simulink library "motohawk_engine_lib"  (Simulink 6.3)
undefined symbols (not defined in the file or in its folder): cast_val, IndPowerMax, InjSequence, lookup_group, MAF_Sensor_p, motohawk_tex, motohawk_vardec_config_group, motohawk_vardec_path, SampleTime, SparkSequence, SteadyStateECT, txtTitle, WarmUpTimeConst
libraries: MotoHawk_lib x234, motohawk_annotations_lib x22, motohawk_control_primitives_lib x20, motohawk_engine_lib x8, motohawk_control_primitives_lib_new x3
(part 7 of 7)

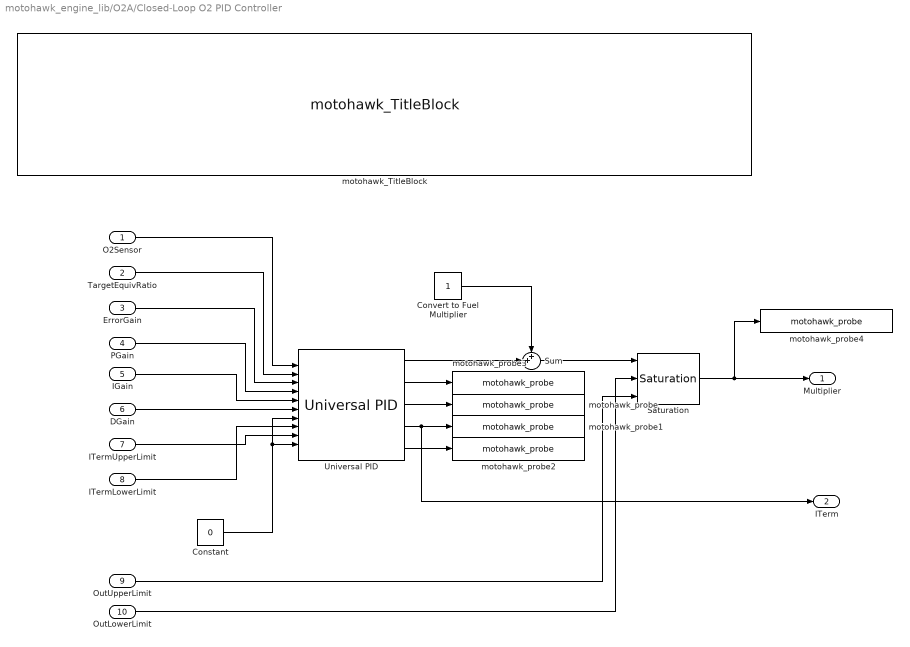
== system motohawk_engine_lib/O2A/Closed-Loop O2 PID Controller ==
  O2Sensor : Inport
  TargetEquivRatio : Inport  Port=2
  ErrorGain : Inport  Port=3
  PGain : Inport  Port=4
  IGain : Inport  Port=5
  DGain : Inport  Port=6
  ITermUpperLimit : Inport  Port=7
  ITermLowerLimit : Inport  Port=8
  OutUpperLimit : Inport  Port=9
  OutLowerLimit : Inport  Port=10
  Constant : Constant  Value=0
  Convert to Fuel Multiplier : Constant
  Saturation : motohawk_control_primitives_lib/Saturation
  Sum : Sum  Inputs=++|  SaturateOnIntegerOverflow=on  InputSameDT=on
  Universal PID : motohawk_control_primitives_lib/Universal PID  Description=|  samp_time=-1
      | /* Name: ErrorGain Unit:mult ClassID:VAR StorageID:FLASH Access:RW4+RW3+NA2+NA1 TypeID:UINT4                   
      |    Gain:0.000000001 Min:0.000000000 Max:4.000000000 Format:10.9 UpdateID:REMOTE Help:"This gain is applied to "
      |    "the error term before it is used to calculate the P, I and D terms." VardecSig:6C */                       
      |                                                                                                                
      | /* Name: ITermLowerLim Unit:0 ClassID:VAR StorageID:FLASH Access:RW4+RW3+NA2+NA1 TypeID:SINT2 Gain:0.1         
      |    Min:-3276.8 Max:3276.7 Format:5.1 UpdateID:REMOTE Help:"Lower limit on the I-term value." VardecSig:6C */   
      |                                                                                                                
      | /* Name: ITermUpperLim ClassID:VAR StorageID:FLASH Access:RW4+RW3+NA2+NA1 TypeID:SINT2 Gain:0.1 Min:-3276.8    
      |    Max:3276.7 Format:5.1 UpdateID:REMOTE Help:"Upper limit on I-term value." VardecSig:6C */                   
      |                                                                                                                
      | /* Name: PIDOutLowerLim ClassID:VAR StorageID:FLASH Access:RW4+RW3+NA2+NA1 TypeID:SINT2 Gain:0.1               
      |    Min:-3276.8 Max:3276.7 Format:5.1 UpdateID:REMOTE Help:"Lower limit on PID output." VardecSig:6C */         
      |                                                                                                                
      | /* Name: PIDOutUpperLim ClassID:VAR StorageID:FLASH Access:RW4+RW3+NA2+NA1 TypeID:SINT2 Gain:0.1               
      |    Min:-3276.8 Max:3276.7 Format:3.1 UpdateID:REMOTE Help:"Upper limit on PID output." VardecSig:6C */
  motohawk_TitleBlock : motohawk_annotations_lib/motohawk_TitleBlock  BlockType_='Mototron_Title_Block'  ttl=[txtTitle '\newline\rmClosed-loop O2 Control - PID for Bank A']  copyright="'THE INFORMATION CONTAINED IN THIS\\newlineDRAWING IS THE SOLE PROPERTY OF\\newlineMOTOTRON.  ANY REPRODUCTION IN\\newline PART OR AS A WHOLE WITHOUT THE\\newlineWRITTEN PERMISSION OF MOTOTRON\\newline IS PROHIBITED.\\fontsize{16}\\rm\\copyright\\rm\\fontsize{10} 2005'"  address='\fontsize{22}\it\fontname{Arial Black}MotoTron Corporation \fontname{Arial}\fontsize{10}\newline505 Marion Road, Oshkosh, WI, 54901\newlinewww.mototron.com (734) 822-7700'  image_file='mh.jpg'  pretty_print=on  edit_text=[motohawk_tex(get_param(bdroot, 'Description')) '\rm\newline' motohawk_tex(get_param(gcs, 'Name'))]  edit_as=6
  motohawk_probe : MotoHawk_lib/Calibration & Probing Blocks/motohawk_probe  nam=['O2Control_PTerm' bank]  show_more=on  name_source=Use Parameter  read_level=1  view_as=Number  enum_struct={'Disabled', 'Enabled'}  vector_style=Wide Row  use_help_units=on  help=['Closed-loop O2 control P-Term, for bank ' bank]  units='mult'  use_header_enum=off  row_header_enum={}  col_header_enum={}  use_precision=off  precision=''  gain=1  offset=0  exp=1  use_mototune_group=on  mototune_group=display_group
  motohawk_probe1 : MotoHawk_lib/Calibration & Probing Blocks/motohawk_probe  nam=['O2Control_ITerm' bank]  show_more=on  name_source=Use Parameter  read_level=1  view_as=Number  enum_struct={'Disabled', 'Enabled'}  vector_style=Wide Row  use_help_units=on  help=['Closed-loop O2 control I-Term, for bank ' bank]  units='mult'  use_header_enum=off  row_header_enum={}  col_header_enum={}  use_precision=off  precision=''  gain=1  offset=0  exp=1  use_mototune_group=on  mototune_group=display_group
  motohawk_probe2 : MotoHawk_lib/Calibration & Probing Blocks/motohawk_probe  nam=['O2Control_DTerm' bank]  show_more=on  name_source=Use Parameter  read_level=1  view_as=Number  enum_struct={'Disabled', 'Enabled'}  vector_style=Wide Row  use_help_units=on  help=['Closed-loop O2 control D-Term, for bank ' bank]  units='mult'  use_header_enum=off  row_header_enum={}  col_header_enum={}  use_precision=off  precision=''  gain=1  offset=0  exp=1  use_mototune_group=on  mototune_group=display_group
  motohawk_probe3 : MotoHawk_lib/Calibration & Probing Blocks/motohawk_probe  nam=['O2Control_ErrorTerm' bank]  show_more=on  name_source=Use Parameter  read_level=1  view_as=Number  enum_struct={'Disabled', 'Enabled'}  vector_style=Wide Row  use_help_units=on  help=['Closed-loop O2 control error-term, for bank ' bank]  units='mult'  use_header_enum=off  row_header_enum={}  col_header_enum={}  use_precision=off  precision=''  gain=1  offset=0  exp=1  use_mototune_group=on  mototune_group=display_group
  motohawk_probe4 : MotoHawk_lib/Calibration & Probing Blocks/motohawk_probe  nam=['O2FuelMult' bank]  show_more=on  name_source=Use Parameter  read_level=1  view_as=Number  enum_struct={'Disabled', 'Enabled'}  vector_style=Wide Row  use_help_units=on  help=['Closed-loop O2 control fuel multiplier, for bank ' bank]  units='mult'  use_header_enum=off  row_header_enum={}  col_header_enum={}  use_precision=off  precision=''  gain=1  offset=0  exp=1  use_mototune_group=on  mototune_group=display_group
  Multiplier : Outport
  ITerm : Outport  Port=2
  wires:
  Universal PID/2 -> motohawk_probe3/1
  OutLowerLimit/1 -> Saturation/2
  ITermLowerLimit/1 -> Universal PID/8
  ITermUpperLimit/1 -> Universal PID/9
  Sum/1 -> Saturation/1
  Universal PID/1 -> Sum/2
  Convert to Fuel Multiplier/1 -> Sum/1
  OutUpperLimit/1 -> Saturation/3
  DGain/1 -> Universal PID/6
  IGain/1 -> Universal PID/5
  PGain/1 -> Universal PID/4
  ErrorGain/1 -> Universal PID/3
  TargetEquivRatio/1 -> Universal PID/2
  O2Sensor/1 -> Universal PID/1
  Saturation/1 -> motohawk_probe4/1, Multiplier/1
  Universal PID/5 -> motohawk_probe2/1
  Constant/1 -> Universal PID/7, Universal PID/10
  Universal PID/4 -> ITerm/1, motohawk_probe1/1
  Universal PID/3 -> motohawk_probe/1

== system motohawk_engine_lib/O2A/Equivalence Ratio Perturbation ==
  note: When low, switch to rich.
      | When high, switch to lean.
  O2Sensor : Inport
  DesEquivRatio : Inport  Port=2
  RichEquivRatioTargetDelta : Inport  Port=3
  LeanEquivRatioTargetDelta : Inport  Port=4
  RichEquivRatioSwPtDelta : Inport  Port=5
  LeanEquivRatioSwPtDelta : Inport  Port=6
  Hysteresis : Subsystem
  LT : RelationalOperator  ZeroCross=off  InputSameDT=on
  LT1 : RelationalOperator  Operator=<=  ZeroCross=off  InputSameDT=on
  Logical Operator : Logic  Operator=NOT
  Sum1 : Sum  SaturateOnIntegerOverflow=on
  Sum2 : Sum  Inputs=-+  SaturateOnIntegerOverflow=on
  Sum3 : Sum  SaturateOnIntegerOverflow=on
  Sum4 : Sum  Inputs=+-  SaturateOnIntegerOverflow=on
  Switch2 : Switch  Threshold=1  ZeroCross=off  InputSameDT=on
  motohawk_TitleBlock : motohawk_annotations_lib/motohawk_TitleBlock  BlockType_='Mototron_Title_Block'  ttl=[txtTitle '\newline\rmO2 Control Target Equivalence Ratio Perturbation around Stoichiometric']  copyright="'THE INFORMATION CONTAINED IN THIS\\newlineDRAWING IS THE SOLE PROPERTY OF\\newlineMOTOTRON.  ANY REPRODUCTION IN\\newline PART OR AS A WHOLE WITHOUT THE\\newlineWRITTEN PERMISSION OF MOTOTRON\\newline IS PROHIBITED.\\fontsize{16}\\rm\\copyright\\rm\\fontsize{10} 2005'"  address='\fontsize{22}\it\fontname{Arial Black}MotoTron Corporation \fontname{Arial}\fontsize{10}\newline505 Marion Road, Oshkosh, WI, 54901\newlinewww.mototron.com (734) 822-7700'  image_file='mh.jpg'  pretty_print=on  edit_text=[motohawk_tex(get_param(bdroot, 'Description')) '\rm\newline' motohawk_tex(get_param(gcs, 'Name'))]  edit_as=6
  motohawk_fault_def : MotoHawk_lib/Fault Management Blocks/motohawk_fault_def  nam=['O2FailedLean',bank]  mode=Enabled  id=[]  x=25  y=50  input_suspected=on  indeterminate=off  increment_xy=on  downsample_count=1  ovr_cals=on  ovr_actions=on  show_actions=off  action1_name=''  action1_cond=(None)  action2_name=''  action2_cond=(None)  action3_name=''  action3_cond=(None)  action4_name=''  action4_cond=(None)
  motohawk_fault_def1 : MotoHawk_lib/Fault Management Blocks/motohawk_fault_def  nam=['O2FailedRich',bank]  mode=Enabled  id=[]  x=25  y=50  input_suspected=on  indeterminate=off  increment_xy=on  downsample_count=1  ovr_cals=on  ovr_actions=on  show_actions=off  action1_name=''  action1_cond=(None)  action2_name=''  action2_cond=(None)  action3_name=''  action3_cond=(None)  action4_name=''  action4_cond=(None)
  Target Phi : Outport
  wires:
  Logical Operator/1 -> Switch2/2
  O2Sensor/1 -> LT/1, LT1/1
  Hysteresis/1("Out (Lo=0, Hi=1)") -> Logical Operator/1
  LT1/1 -> motohawk_fault_def/1, Hysteresis/2(Lo)  "BelowLean"
  LT/1 -> motohawk_fault_def1/1, Hysteresis/1(Hi)  "AboveRich"
  RichEquivRatioTargetDelta/1 -> Sum1/1
  LeanEquivRatioTargetDelta/1 -> Sum2/1
  Sum1/1 -> Switch2/1
  Sum2/1 -> Switch2/3
  LeanEquivRatioSwPtDelta/1 -> Sum4/2
  RichEquivRatioSwPtDelta/1 -> Sum3/2
  DesEquivRatio/1 -> Sum3/1, Sum4/1, Sum2/2, Sum1/2
  Switch2/1 -> Target Phi/1
  Sum4/1 -> LT1/2
  Sum3/1 -> LT/2

== system motohawk_engine_lib/O2A/O2 Calibrations ==
  Bus Creator : BusCreator  Inputs=12
  motohawk_TitleBlock : motohawk_annotations_lib/motohawk_TitleBlock  BlockType_='Mototron_Title_Block'  ttl=[txtTitle '\newline\rmClosed-Loop O2 Control Calibrations']  copyright="'THE INFORMATION CONTAINED IN THIS\\newlineDRAWING IS THE SOLE PROPERTY OF\\newlineMOTOTRON.  ANY REPRODUCTION IN\\newline PART OR AS A WHOLE WITHOUT THE\\newlineWRITTEN PERMISSION OF MOTOTRON\\newline IS PROHIBITED.\\fontsize{16}\\rm\\copyright\\rm\\fontsize{10} 2005'"  address='\fontsize{22}\it\fontname{Arial Black}MotoTron Corporation \fontname{Arial}\fontsize{10}\newline505 Marion Road, Oshkosh, WI, 54901\newlinewww.mototron.com (734) 822-7700'  image_file='mh.jpg'  pretty_print=on  edit_text=[motohawk_tex(get_param(bdroot, 'Description')) '\rm\newline' motohawk_tex(get_param(gcs, 'Name'))]  edit_as=6
  motohawk_calibration1 : MotoHawk_lib/Calibration & Probing Blocks/motohawk_calibration  nam=['LeanEquivRatioTargetDelta' bank]  val=.05  storage=Calibration  show_more=on  name_source=Use Parameter  data_type=Inherit from 'Default Value'  read_level=1  write_level=1  ovr_cals=on  view_as=Number  enum_struct={'Disabled', 'Enabled'}  vector_style=Wide Row  use_help_units=on  help='Target equivalence ratio below desired, when driving lean'  units='ratio'  use_header_enum=off  row_header_enum={}  col_header_enum={}  use_min_max=on  min_val=0  max_val=1.0  use_precision=off  precision=''  gain=1  offset=0  exp=1  use_mototune_group=on  mototune_group=cal_group
  motohawk_calibration10 : MotoHawk_lib/Calibration & Probing Blocks/motohawk_calibration  nam=['O2ControlOutUpperLimit',bank]  val=1.4  storage=Calibration  show_more=on  name_source=Use Parameter  data_type=Inherit from 'Default Value'  read_level=1  write_level=1  ovr_cals=on  view_as=Number  enum_struct={'Disabled', 'Enabled'}  vector_style=Wide Row  use_help_units=on  help='PID fuel multiplier output upper limit for closed-loop O2 control'  units='mult'  use_header_enum=off  row_header_enum={}  col_header_enum={}  use_min_max=on  min_val=-inf  max_val=inf  use_precision=off  precision=''  gain=1  offset=0  exp=1  use_mototune_group=on  mototune_group=cal_group
  motohawk_calibration11 : MotoHawk_lib/Calibration & Probing Blocks/motohawk_calibration  nam=['O2ControlOutLowerLimit',bank]  val=.6  storage=Calibration  show_more=on  name_source=Use Parameter  data_type=Inherit from 'Default Value'  read_level=1  write_level=1  ovr_cals=on  view_as=Number  enum_struct={'Disabled', 'Enabled'}  vector_style=Wide Row  use_help_units=on  help='PID fuel multiplier output lower limit for closed-loop O2 control'  units='mult'  use_header_enum=off  row_header_enum={}  col_header_enum={}  use_min_max=on  min_val=-inf  max_val=inf  use_precision=off  precision=''  gain=1  offset=0  exp=1  use_mototune_group=on  mototune_group=cal_group
  motohawk_calibration12 : MotoHawk_lib/Calibration & Probing Blocks/motohawk_calibration  nam=['RichEquivRatioTargetDelta' bank]  val=.05  storage=Calibration  show_more=on  name_source=Use Parameter  data_type=Inherit from 'Default Value'  read_level=1  write_level=1  ovr_cals=on  view_as=Number  enum_struct={'Disabled', 'Enabled'}  vector_style=Wide Row  use_help_units=on  help='Target equivalence ratio below desired, when driving lean'  units='ratio'  use_header_enum=off  row_header_enum={}  col_header_enum={}  use_min_max=on  min_val=0  max_val=1.0  use_precision=off  precision=''  gain=1  offset=0  exp=1  use_mototune_group=on  mototune_group=cal_group
  motohawk_calibration2 : MotoHawk_lib/Calibration & Probing Blocks/motohawk_calibration  nam=['RichEquivRatioSwPtDelta',bank]  val=.01  storage=Calibration  show_more=on  name_source=Use Parameter  data_type=Inherit from 'Default Value'  read_level=1  write_level=1  ovr_cals=on  view_as=Number  enum_struct={'Disabled', 'Enabled'}  vector_style=Wide Row  use_help_units=on  help='Switch point equivalence ratio above desired, when driving rich, and changing to lean'  units='ratio'  use_header_enum=off  row_header_enum={}  col_header_enum={}  use_min_max=on  min_val=0  max_val=1.0  use_precision=off  precision=''  gain=1  offset=0  exp=1  use_mototune_group=on  mototune_group=cal_group
  motohawk_calibration3 : MotoHawk_lib/Calibration & Probing Blocks/motohawk_calibration  nam=['LeanEquivRatioSwPtDelta',bank]  val=.01  storage=Calibration  show_more=on  name_source=Use Parameter  data_type=Inherit from 'Default Value'  read_level=1  write_level=1  ovr_cals=on  view_as=Number  enum_struct={'Disabled', 'Enabled'}  vector_style=Wide Row  use_help_units=on  help='Switch point equivalence ratio below desired, when driving lean, and changing to rich'  units='ratio'  use_header_enum=off  row_header_enum={}  col_header_enum={}  use_min_max=on  min_val=0  max_val=1.0  use_precision=off  precision=''  gain=1  offset=0  exp=1  use_mototune_group=on  mototune_group=cal_group
  motohawk_calibration4 : MotoHawk_lib/Calibration & Probing Blocks/motohawk_calibration  nam=['O2ControlErrorGain',bank]  val=.2  storage=Calibration  show_more=on  name_source=Use Parameter  data_type=Inherit from 'Default Value'  read_level=1  write_level=1  ovr_cals=on  view_as=Number  enum_struct={'Disabled', 'Enabled'}  vector_style=Wide Row  use_help_units=on  help='PID error gain for closed-loop O2 control'  units='mult'  use_header_enum=off  row_header_enum={}  col_header_enum={}  use_min_max=on  min_val=-inf  max_val=inf  use_precision=off  precision=''  gain=1  offset=0  exp=1  use_mototune_group=on  mototune_group=cal_group
  motohawk_calibration5 : MotoHawk_lib/Calibration & Probing Blocks/motohawk_calibration  nam=['O2ControlPGain',bank]  val=1  storage=Calibration  show_more=on  name_source=Use Parameter  data_type=Inherit from 'Default Value'  read_level=1  write_level=1  ovr_cals=on  view_as=Number  enum_struct={'Disabled', 'Enabled'}  vector_style=Wide Row  use_help_units=on  help='PID P-Term gain for closed-loop O2 control'  units='mult'  use_header_enum=off  row_header_enum={}  col_header_enum={}  use_min_max=on  min_val=-inf  max_val=inf  use_precision=off  precision=''  gain=1  offset=0  exp=1  use_mototune_group=on  mototune_group=cal_group
  motohawk_calibration6 : MotoHawk_lib/Calibration & Probing Blocks/motohawk_calibration  nam=['O2ControlIGain',bank]  val=2  storage=Calibration  show_more=on  name_source=Use Parameter  data_type=Inherit from 'Default Value'  read_level=1  write_level=1  ovr_cals=on  view_as=Number  enum_struct={'Disabled', 'Enabled'}  vector_style=Wide Row  use_help_units=on  help='PID I-Term gain for closed-loop O2 control'  units='mult'  use_header_enum=off  row_header_enum={}  col_header_enum={}  use_min_max=on  min_val=-inf  max_val=inf  use_precision=off  precision=''  gain=1  offset=0  exp=1  use_mototune_group=on  mototune_group=cal_group
  motohawk_calibration7 : MotoHawk_lib/Calibration & Probing Blocks/motohawk_calibration  nam=['O2ControlDGain',bank]  val=0  storage=Calibration  show_more=on  name_source=Use Parameter  data_type=Inherit from 'Default Value'  read_level=1  write_level=1  ovr_cals=on  view_as=Number  enum_struct={'Disabled', 'Enabled'}  vector_style=Wide Row  use_help_units=on  help='PID D-Term gain for closed-loop O2 control'  units='mult'  use_header_enum=off  row_header_enum={}  col_header_enum={}  use_min_max=on  min_val=-inf  max_val=inf  use_precision=off  precision=''  gain=1  offset=0  exp=1  use_mototune_group=on  mototune_group=cal_group
  motohawk_calibration8 : MotoHawk_lib/Calibration & Probing Blocks/motohawk_calibration  nam=['O2ControlITermLowerLimit',bank]  val=-.4  storage=Calibration  show_more=on  name_source=Use Parameter  data_type=Inherit from 'Default Value'  read_level=1  write_level=1  ovr_cals=on  view_as=Number  enum_struct={'Disabled', 'Enabled'}  vector_style=Wide Row  use_help_units=on  help='PID I-Term lower limit for closed-loop O2 control'  units='mult'  use_header_enum=off  row_header_enum={}  col_header_enum={}  use_min_max=on  min_val=-inf  max_val=inf  use_precision=off  precision=''  gain=1  offset=0  exp=1  use_mototune_group=on  mototune_group=cal_group
  motohawk_calibration9 : MotoHawk_lib/Calibration & Probing Blocks/motohawk_calibration  nam=['O2ControlITermUpperLimit',bank]  val=.3  storage=Calibration  show_more=on  name_source=Use Parameter  data_type=Inherit from 'Default Value'  read_level=1  write_level=1  ovr_cals=on  view_as=Number  enum_struct={'Disabled', 'Enabled'}  vector_style=Wide Row  use_help_units=on  help='PID I-Term upper limit for closed-loop O2 control'  units='mult'  use_header_enum=off  row_header_enum={}  col_header_enum={}  use_min_max=on  min_val=-inf  max_val=inf  use_precision=off  precision=''  gain=1  offset=0  exp=1  use_mototune_group=on  mototune_group=cal_group
  Calibrations : Outport
  wires:
  motohawk_calibration12/1 -> Bus Creator/1  "RichEquivRatioTargetDelta"
  Bus Creator/1 -> Calibrations/1
  motohawk_calibration11/1 -> Bus Creator/12  "O2ControlOutLowerLimit"
  motohawk_calibration10/1 -> Bus Creator/11  "O2ControlOutUpperLimit"
  motohawk_calibration8/1 -> Bus Creator/10  "O2ControlItermLowerLimit"
  motohawk_calibration9/1 -> Bus Creator/9  "O2ControlITermUpperLimit"
  motohawk_calibration7/1 -> Bus Creator/8  "O2ControlDGain"
  motohawk_calibration6/1 -> Bus Creator/7  "O2ControlIGain"
  motohawk_calibration5/1 -> Bus Creator/6  "O2ControlPGain"
  motohawk_calibration4/1 -> Bus Creator/5  "O2ControlErrorGain"
  motohawk_calibration3/1 -> Bus Creator/4  "LeanEquivRatioSwPtDelta"
  motohawk_calibration2/1 -> Bus Creator/3  "RichEquivRatioSwPtDelta"
  motohawk_calibration1/1 -> Bus Creator/2  "LeanEquivRatioTargetDelta"

== system motohawk_engine_lib/Speed Density - MAP Referenced/C to K1 ==
  C : Inport
  C to K : Fcn  Expr=u(1) + 273.2
  K : Outport
  wires:
  C/1 -> C to K/1
  C to K/1 -> K/1

== system motohawk_engine_lib/Speed Density - MAP Referenced - Adaptive/Adapt Volumetric Efficiency ==
  SSEngOpr [bool] : Inport
  MAF_Sensor [g/s] : Inport  Port=2
  MAF_Model [g/s] : Inport  Port=3
  Abs : Abs  SaturateOnIntegerOverflow=on
  Adapt VolEff Map : Subsystem
  Logical Operator : Logic  Inputs=3
  Product0 : Product  SaturateOnIntegerOverflow=on  InputSameDT=on
  Relational Operator : RelationalOperator  Operator=<=  InputSameDT=on
  Safe Divide : Subsystem
  Sum1 : Sum  Inputs=+-  SaturateOnIntegerOverflow=on  InputSameDT=on
  motohawk_TitleBlock : motohawk_annotations_lib/motohawk_TitleBlock  BlockType_='Mototron_Title_Block'  ttl=[txtTitle '\newline\rmDetermine whether to adapt the volumetric efficiency map\newlineand compute the error for modifying the map']  copyright="'THE INFORMATION CONTAINED IN THIS\\newlineDRAWING IS THE SOLE PROPERTY OF\\newlineMOTOTRON.  ANY REPRODUCTION IN\\newline PART OR AS A WHOLE WITHOUT THE\\newlineWRITTEN PERMISSION OF MOTOTRON\\newline IS PROHIBITED.\\fontsize{16}\\rm\\copyright\\rm\\fontsize{10} 2005'"  address='\fontsize{22}\it\fontname{Arial Black}MotoTron Corporation \fontname{Arial}\fontsize{10}\newline505 Marion Road, Oshkosh, WI, 54901\newlinewww.mototron.com (734) 822-7700'  image_file='mh.jpg'  pretty_print=on  edit_text=[motohawk_tex(get_param(bdroot, 'Description')) '\rm\newline' motohawk_tex(get_param(gcs, 'Name'))]  edit_as=6
  motohawk_calibration : MotoHawk_lib/Calibration & Probing Blocks/motohawk_calibration  nam='VEAdaptEnable'  val=false  storage=Display  show_more=on  name_source=Use Parameter  data_type=Inherit from 'Default Value'  read_level=1  write_level=1  ovr_cals=on  view_as=Enumeration  enum_struct={'Disabled', 'Enabled'}  vector_style=Wide Row  use_help_units=on  help='Determines whether the Volumetric Efficiency map will be adapted using the MAF sensor'  units='bool'  use_header_enum=off  row_header_enum={}  col_header_enum={}  use_min_max=off  min_val=-inf  max_val=inf  use_precision=off  precision=''  gain=1  offset=0  exp=1  use_mototune_group=on  mototune_group=lookup_group(gcb)
  motohawk_calibration1 : MotoHawk_lib/Calibration & Probing Blocks/motohawk_calibration  nam='VEAdaptDelta'  val=VEAdaptDelta  storage=Calibration  show_more=on  name_source=Use Parameter  data_type=Inherit from 'Default Value'  read_level=1  write_level=1  ovr_cals=on  view_as=Number  enum_struct={'Disabled', 'Enabled'}  vector_style=Wide Row  use_help_units=on  help='VolEff_Error must be less than this delta to adapt the VolEff map'  units='mult'  use_header_enum=off  row_header_enum={}  col_header_enum={}  use_min_max=on  min_val=0  max_val=2  use_precision=off  precision=''  gain=1  offset=0  exp=1  use_mototune_group=on  mototune_group=lookup_group(gcb)
  motohawk_calibration2 : MotoHawk_lib/Calibration & Probing Blocks/motohawk_calibration  nam='VEAdaptGain'  val=VEAdaptGain  storage=Calibration  show_more=on  name_source=Use Parameter  data_type=Inherit from 'Default Value'  read_level=1  write_level=1  ovr_cals=on  view_as=Number  enum_struct={'Disabled', 'Enabled'}  vector_style=Wide Row  use_help_units=on  help="'Gain for updating VE table.  This fraction of the error is added to the map every 5ms.'"  units=''  use_header_enum=off  row_header_enum={}  col_header_enum={}  use_min_max=on  min_val=0  max_val=1  use_precision=off  precision='8.6'  gain=1  offset=0  exp=1  use_mototune_group=on  mototune_group=lookup_group(gcb)
  motohawk_probe1 : MotoHawk_lib/Calibration & Probing Blocks/motohawk_probe  nam='VolEff_Error'  show_more=on  name_source=Use Parameter  read_level=1  view_as=Number  enum_struct={'Disabled', 'Enabled'}  vector_style=Wide Row  use_help_units=on  help='Error in Volumetric Efficiency at the current operating point, as compared to MAF sensor'  units=''  use_header_enum=off  row_header_enum={}  col_header_enum={}  use_precision=off  precision=''  gain=1  offset=0  exp=1  use_mototune_group=on  mototune_group=lookup_group(gcb)
  motohawk_probe2 : MotoHawk_lib/Calibration & Probing Blocks/motohawk_probe  nam='MAF_ModelError'  show_more=on  name_source=Use Parameter  read_level=1  view_as=Number  enum_struct={'Disabled', 'Enabled'}  vector_style=Wide Row  use_help_units=on  help='Air Mass Flow Rate error, as compared to MAF sensor'  units='g/s'  use_header_enum=off  row_header_enum={}  col_header_enum={}  use_precision=off  precision=''  gain=1  offset=0  exp=1  use_mototune_group=on  mototune_group=lookup_group(gcb)
  motohawk_probe3 : MotoHawk_lib/Calibration & Probing Blocks/motohawk_probe  nam='VEAdapting'  show_more=on  name_source=Use Parameter  read_level=1  view_as=Enumeration  enum_struct={'Not adapting', 'Adapting'}  vector_style=Wide Row  use_help_units=on  help='Indicates whether the volumetric efficiency map is currently being adjusted'  units=''  use_header_enum=off  row_header_enum={}  col_header_enum={}  use_precision=off  precision=''  gain=1  offset=0  exp=1  use_mototune_group=on  mototune_group=lookup_group(gcb)
  wires:
  Product0/1 -> Adapt VolEff Map/1(error)
  motohawk_calibration2/1 -> Product0/2
  MAF_Model [g/s]/1 -> Safe Divide/2(Inport), Sum1/2
  MAF_Sensor [g/s]/1 -> Sum1/1
  Sum1/1 -> Safe Divide/1(X), motohawk_probe2/1
  Safe Divide/1(" ") -> Abs/1, motohawk_probe1/1, Product0/1
  motohawk_calibration1/1 -> Relational Operator/2
  Relational Operator/1 -> Logical Operator/3
  Abs/1 -> Relational Operator/1
  SSEngOpr [bool]/1 -> Logical Operator/2
  Logical Operator/1 -> motohawk_probe3/1, Adapt VolEff Map/Enable
  motohawk_calibration/1 -> Logical Operator/1

== system motohawk_engine_lib/Speed Density - MAP Referenced - Adaptive/C to K1 ==
  C : Inport
  C to K : Fcn  Expr=u(1) + 273.2
  K : Outport
  wires:
  C to K/1 -> K/1
  C/1 -> C to K/1

== system motohawk_engine_lib/Subsystem/Enabled Subsystem ==
  In1 : Inport
  Enable : EnablePort  StatesWhenEnabling=reset
  Out1 : Outport  OutputWhenDisabled=reset  InitialOutput=0
  wires:
  In1/1 -> Out1/1

== system motohawk_engine_lib/Idle Governor/Idle State Determination/Determine if RPM is Falling ==
  note: Determine whether RPM is falling
  RPM : Inport
  Derivitive : motohawk_control_primitives_lib/Derivitive  samp_time=-1
  Falling RPM is Negative Derivative : Gain  Gain=-1
  Median Filter : motohawk_control_primitives_lib/Median Filter  buffer_size=17
  Relational Operator : RelationalOperator  Operator=<
  motohawk_calibration : MotoHawk_lib/Calibration & Probing Blocks/motohawk_calibration  nam='RPMFallingRate'  val=4  storage=Calibration  show_more=on  name_source=Use Parameter  data_type=Inherit from 'Default Value'  read_level=1  write_level=1  ovr_cals=on  view_as=Number  enum_struct={'Disabled', 'Enabled'}  vector_style=Wide Row  use_help_units=on  help='The minimum rate of change in RPM that triggers RPMFalling - This should be a positive value'  units='RPM/sec'  use_header_enum=off  row_header_enum={}  col_header_enum={}  use_min_max=on  min_val=0  max_val=1000  use_precision=off  precision=''  gain=1  offset=0  exp=1  use_mototune_group=off  mototune_group=motohawk_vardec_path(gcb)
  motohawk_probe : MotoHawk_lib/Calibration & Probing Blocks/motohawk_probe  nam='RPMFalling'  show_more=off  name_source=Use Parameter  read_level=1  view_as=Number  enum_struct={'Disabled', 'Enabled'}  vector_style=Wide Row  use_help_units=off  help=''  units=''  use_header_enum=off  row_header_enum={}  col_header_enum={}  use_precision=off  precision=''  gain=1  offset=0  exp=1  use_mototune_group=off  mototune_group=motohawk_vardec_path(gcb)
  RPM Falling : Outport
  wires:
  Falling RPM is Negative Derivative/1 -> Relational Operator/2
  RPM/1 -> Derivitive/1
  Relational Operator/1 -> RPM Falling/1, motohawk_probe/1
  motohawk_calibration/1 -> Falling RPM is Negative Derivative/1
  Median Filter/1 -> Relational Operator/1
  Derivitive/1 -> Median Filter/1

== system motohawk_engine_lib/Linear Sensor Characterization w Adapt/ADAPT SCALING/ADAPT HI ==
  ADAPT_REQUEST : Inport
  ADAPT_ENABLE : Inport  Port=2
  CUR_ADAPT_PT : Inport  Port=3
  ADAPT_RANGE_MAX : Inport  Port=4
  ADAPT_RANGE_MIN : Inport  Port=5
  ADAPT_MIN_DELTA : Inport  Port=6
  MAX_LAST5 : Inport  Port=7
  Abs : Abs  SaturateOnIntegerOverflow=on
  Data Type Conversion : DataTypeConversion  OutDataTypeMode=double  SaturateOnIntegerOverflow=on  RndMeth=Zero
  Logical Operator1 : Logic  Inputs=5  AllPortsSameDT=off
  Logical Operator2 : Logic  Operator=OR  AllPortsSameDT=off
  Logical Operator4 : Logic  Inputs=4  AllPortsSameDT=off
  Relational Operator3 : RelationalOperator  Operator=>  LogicOutDataTypeMode=Boolean
  Relational Operator5 : RelationalOperator  Operator=<=  LogicOutDataTypeMode=Boolean
  Relational Operator6 : RelationalOperator  LogicOutDataTypeMode=Boolean
  Relational Operator9 : RelationalOperator  Operator=>  LogicOutDataTypeMode=Boolean
  Store Current Position : Subsystem  TreatAsAtomicUnit=on
  Sum2 : Sum  Inputs=|+-  SaturateOnIntegerOverflow=on
  ADAPTED_ENDPT : Outport
  wires:
  ADAPT_REQUEST/1 -> Logical Operator4/4
  Logical Operator4/1 -> Logical Operator2/2
  MAX_LAST5/1 -> Relational Operator6/1, Relational Operator5/1, Relational Operator9/1, Store Current Position/1(IN_FILT), Sum2/1
  ADAPT_ENABLE/1 -> Logical Operator4/3, Logical Operator1/4
  Data Type Conversion/1 -> Sum2/2, Relational Operator9/2, ADAPTED_ENDPT/1
  ADAPT_MIN_DELTA/1 -> Relational Operator3/2
  Abs/1 -> Relational Operator3/1
  Relational Operator3/1 -> Logical Operator1/5
  Sum2/1 -> Abs/1
  CUR_ADAPT_PT/1 -> Data Type Conversion/1
  Relational Operator9/1 -> Logical Operator1/1
  Relational Operator5/1 -> Logical Operator4/1, Logical Operator1/2
  Relational Operator6/1 -> Logical Operator4/2, Logical Operator1/3
  ADAPT_RANGE_MAX/1 -> Relational Operator5/2
  ADAPT_RANGE_MIN/1 -> Relational Operator6/2
  Logical Operator1/1 -> Logical Operator2/1
  Logical Operator2/1 -> Store Current Position/Enable

== system motohawk_engine_lib/Linear Sensor Characterization w Adapt/ADAPT SCALING/ADAPT LO ==
  ADAPT_REQUEST : Inport
  ADAPT_ENABLE : Inport  Port=2
  CUR_ADAPT_PT : Inport  Port=3
  ADAPT_RANGE_MAX : Inport  Port=4
  ADAPT_RANGE_MIN : Inport  Port=5
  ADAPT_MIN_DELTA : Inport  Port=6
  MAX_LAST5 : Inport  Port=7
  Abs : Abs  SaturateOnIntegerOverflow=on
  Data Type Conversion : DataTypeConversion  OutDataTypeMode=double  SaturateOnIntegerOverflow=on  RndMeth=Zero
  Logical Operator1 : Logic  Inputs=5  AllPortsSameDT=off
  Logical Operator2 : Logic  Operator=OR  AllPortsSameDT=off
  Logical Operator4 : Logic  Inputs=4  AllPortsSameDT=off
  Relational Operator3 : RelationalOperator  Operator=>  LogicOutDataTypeMode=Boolean
  Relational Operator5 : RelationalOperator  Operator=<=  LogicOutDataTypeMode=Boolean
  Relational Operator6 : RelationalOperator  LogicOutDataTypeMode=Boolean
  Relational Operator9 : RelationalOperator  Operator=<  LogicOutDataTypeMode=Boolean
  Store Current Position : Subsystem  TreatAsAtomicUnit=on
  Sum2 : Sum  Inputs=|+-  SaturateOnIntegerOverflow=on
  ADAPTED_ENDPT : Outport
  wires:
  Logical Operator4/1 -> Logical Operator2/2
  ADAPT_REQUEST/1 -> Logical Operator4/4
  Logical Operator2/1 -> Store Current Position/Enable
  Logical Operator1/1 -> Logical Operator2/1
  ADAPT_RANGE_MIN/1 -> Relational Operator6/2
  ADAPT_RANGE_MAX/1 -> Relational Operator5/2
  Relational Operator6/1 -> Logical Operator4/2, Logical Operator1/3
  Relational Operator5/1 -> Logical Operator4/1, Logical Operator1/2
  Relational Operator9/1 -> Logical Operator1/1
  CUR_ADAPT_PT/1 -> Data Type Conversion/1
  Sum2/1 -> Abs/1
  Relational Operator3/1 -> Logical Operator1/5
  Abs/1 -> Relational Operator3/1
  ADAPT_MIN_DELTA/1 -> Relational Operator3/2
  Data Type Conversion/1 -> ADAPTED_ENDPT/1, Relational Operator9/2, Sum2/2
  ADAPT_ENABLE/1 -> Logical Operator4/3, Logical Operator1/4
  MAX_LAST5/1 -> Sum2/1, Store Current Position/1(IN_FILT), Relational Operator9/1, Relational Operator5/1, Relational Operator6/1

== system motohawk_engine_lib/Linear Sensor Characterization w Adapt/ADAPT SCALING/MinMaxFilter ==
  Input : Inport
  Bus Creator : BusCreator  Inputs=2
  MinMax : MinMax  Function=max  Inputs=5  SaturateOnIntegerOverflow=on  InputSameDT=on
  MinMax1 : MinMax  Inputs=5  SaturateOnIntegerOverflow=on  InputSameDT=on
  Unit Delay{,1,3..4} (4 alike) : UnitDelay  SampleTime=-1
  Min_Max : Outport
  wires:
  Input/1 -> Unit Delay4/1, MinMax/1, MinMax1/5
  MinMax1/1 -> Bus Creator/2  "min_last5"
  MinMax/1 -> Bus Creator/1  "max_last5"
  Unit Delay1/1 -> MinMax1/1, MinMax/5
  Unit Delay/1 -> MinMax1/2, Unit Delay1/1, MinMax/4
  Unit Delay3/1 -> Unit Delay/1, MinMax1/3, MinMax/3
  Unit Delay4/1 -> Unit Delay3/1, MinMax1/4, MinMax/2
  Bus Creator/1 -> Min_Max/1

== system motohawk_engine_lib/Model Fuel Puddle Mass/Enabled Tau-X Algorithm/Tau-X Fuel Model ==
  note: Tau - Puddle evaporation time constant
      | X - Fraction of fuel injected that adds to the puddle
  note: Puddle mass is modeled by integrating
      | the difference between the desired fuel rate
      | and the actual fuel rate
  Fdes [g/s] : Inport
  X [frac] : Inport  Port=2
  Tau [1/s] : Inport  Port=3
  MaxPuddle [mg] : Inport  Port=4
  InitPuddle [mg] : Inport  Port=5
  Can't Have Negative Puddle Mass1 : Constant  Value=0
  Can't have negative puddle mass : Constant  Value=0
  Can't inject negative fuel : MinMax  Function=max  Inputs=2  SaturateOnIntegerOverflow=on  InputSameDT=on
  Compute using grams : Gain  Orientation=left  Gain=1/1000  SaturateOnIntegerOverflow=on
  Initialize puddle mass on first sample : motohawk_control_primitives_lib/First Time
  Integrator : motohawk_control_primitives_lib/Integrator  samp_time=samp_time
  Product : Product  Inputs=*/  SaturateOnIntegerOverflow=on
  Store and report in milligrams : Gain  Gain=1000  SaturateOnIntegerOverflow=on
  Sum1 : Sum  Inputs=+-|  SaturateOnIntegerOverflow=on  InputSameDT=on
  "[1/ (1 - X)] [Fdes - Mpud / T]" : Subsystem
  motohawk_TitleBlock : Subsystem  mask{BlockType_='Mototron_Title_Block', ttl='Tau-X Transient Fueling Model\newline\rmUse parameters Tau and X to predictively model a fuel puddle mass\newlineTake into account evaporation from the puddle when calculating the fuel to inject,\newlineso that transient changes in fueling rate do not cause overly lean or rich burns', im=mh.jpg}
      mask prompts: ttl "Description"; im "Image FIle"
      mask init:
      | set_param(gcb,'BlockType_','''Mototron_Title_Block''')
      | set_param(gcb,'MaskVisibilityString','off,on,on');
      mask Display:
      | image(imread(im),[0.31 0.66 0.31 0.35])
      | 
      | plot([0 0 1 1 0],[0 1 1 0 0])
      | plot([.3 1],[0.65 0.65])
      | plot([.3 .3],[0.1 1.0])
      | plot([0 1],[0.1 0.1])
      | plot([0.91 0.91],[0 0.1])
      | text(1,1,'\fontsize{22}\it\fontname{Arial Black}MotoTron Corporation \fontname{Arial}\fontsize{10}\newline505 Marion Road, Oshkosh, WI, 54901\newlinewww.mototron.com (734) 822-7700','verticalAlignment','Top','horizontalAlignment','Right','texmode','on')
      | text(0.01,1,['\fontsize{14}\it\bfPROPRIETARY\newlineAND CONFIDENTIAL\newline\fontsize{10}
      | THE INFORMATION CONTAINED IN THIS\newline
      | DRAWING IS THE SOLE PROPERTY OF\newline
      | MOTOTRON.  ANY REPRODUCTION IN\newline
      | PART OR AS A WHOLE WITHOUT THE\newline
      | WRITTEN PERMISSION OF MOTOTRON\newline
      | IS PROHIBITED.\fontsize{16}\rm\copyright\rm\fontsize{10} 2004' ],'verticalAlignment','Top','horizontalAlignment','Left','texmode','on')
      | 
      | text(0.9,0,['\fontsize{11}\bfPath: \rm' strrep(motohawk_vardec_path(gcb),'_','\_')],'verticalAlignment','Bottom','horizontalAlignment','Right','texmode','on')
      | text(0.31,0.65,['\fontsize{10}\bfDescription:'],'verticalAlignment','Top','horizontalAlignment','Left','texmode','on')
      | 
      | text(0.31,0.55,['\fontsize{14}\bf' ttl],'verticalAlignment','Top','horizontalAlignment','Left','texmode','on')
      | text(0.99,0,['\fontsize{11}\bfREV: \rm' motohawk_build_version],'verticalAlignment','Bottom','horizontalAlignment','Right','texmode','on')
  Finj [g/s] : Outport
  PuddleMass [mg] : Outport  Port=2
  X_Mult : Outport  Port=3
  Tau_Ofst : Outport  Port=4
  TranFuelMult : Outport  Port=5
  wires:
  Product/1 -> TranFuelMult/1
  "[1/ (1 - X)] [Fdes - Mpud / T]"/3(Tau_Ofst) -> Tau_Ofst/1
  "[1/ (1 - X)] [Fdes - Mpud / T]"/2(X_Mult) -> X_Mult/1
  Can't Have Negative Puddle Mass1/1 -> Can't inject negative fuel/1
  Can't inject negative fuel/1 -> Product/1, Sum1/1, Finj [g/s]/1
  "[1/ (1 - X)] [Fdes - Mpud / T]"/1(Finj [g/s]) -> Can't inject negative fuel/2
  InitPuddle [mg]/1 -> Integrator/3
  Initialize puddle mass on first sample/1 -> Integrator/2
  Can't have negative puddle mass/1 -> Integrator/4
  MaxPuddle [mg]/1 -> Integrator/5
  Integrator/1 -> PuddleMass [mg]/1, Compute using grams/1
  Sum1/1 -> Store and report in milligrams/1
  X [frac]/1 -> "[1/ (1 - X)] [Fdes - Mpud / T]"/2(X [frac])
  Tau [1/s]/1 -> "[1/ (1 - X)] [Fdes - Mpud / T]"/3(Tau [1/s])
  Fdes [g/s]/1 -> Product/2, Sum1/2, "[1/ (1 - X)] [Fdes - Mpud / T]"/1(Fdes [g/s])
  Compute using grams/1 -> "[1/ (1 - X)] [Fdes - Mpud / T]"/4(Mpud [g])
  Store and report in milligrams/1 -> Integrator/1

== system motohawk_engine_lib/Model Fuel Puddle Mass/Enabled Tau-X Algorithm/motohawk_TitleBlock ==

== system motohawk_engine_lib/Normalized Effective Combustion Chamber Temperature/Integrate an offset to ECT  Reset offset when engine is stopped./Integrator ==
  note: Discrete Integrator,
      | with output and state saturation.
  In : Inport  Orientation=left
  Rst : Inport  Port=2
  IC : Inport  Port=3
  Min : Inport  Orientation=left  Port=4
  Max : Inport  Orientation=left  Port=5
  Data Type Conversion : DataTypeConversion  RndMeth=Zero
  Product : Product  Orientation=left  SaturateOnIntegerOverflow=on  InputSameDT=on
  Saturation : Subsystem  Orientation=left  mask(Saturation){}
      mask help: Saturation block.
      mask Display:
      | patch([0 0 1 1], [0 0.075 0.075 0], [230/255 0/255 0/255])
      | patch([0 0 1 1], [0.025 0.05 0.05 0.025], [150/255 0/255 0/255])
      | patch([0 0 1 1], [0 0.025 0.025 0], [0/255 0/255 0/255])
      | 
      | plot([.2 .4 .6 .8], [.2 .2 .9 .9])
  Sum : Sum  Orientation=left  Inputs=++|  SaturateOnIntegerOverflow=on  InputSameDT=on
  Switch1 : Switch  Threshold=1  ZeroCross=off  SaturateOnIntegerOverflow=on  InputSameDT=on
  Unit Delay : UnitDelay  Orientation=left  SampleTime=-1
  motohawk_delta_time : S-Function  Orientation=left  FunctionName=motohawk_sfun_delta_time  Parameters=samp_time, double(init_val)  mask(MotoHawk Delta Time){samp_time=samp_time, init_val=0}
      mask prompts: samp_time "Sample Time"; init_val "Initial Value"
      mask help:
      | Outputs the delta time since the last time this block was called (in seconds).
      |
      | If a positive 'Sample Time' is entered, this constant value will be output every time.  The output data type will be the same as the 'Sample Time' parameter.  In this case, the 'Initial Value' parameter is unused.
      |
      | If a zero or negative 'Sample Time' is entered, the block will calculate the delta time, and the block\ will output 'Initial Value' the first time it is called.
      |
      | Using a constant sample time is more efficient than an inherited sample time, because it does not generate extra code and RAM to dynamically calculate the delta time.
      |
      | Note that the block still runs with inherited sample-time in the Simulink environment, regardless of what is entered.  It is legal to insert a 'wrong' value into the Sample Time (a value that doesn't actually represent the number of seconds between executions), and the block will happily output that value.
      |
      | ---------------------------------------------------------------------
      | Copyright 2004 MotoTron, Inc.  All Rights Reserved.
      mask Display:
      | patch([0 0 1 1], [0 1 1 0], [220/255 220/255 220/255])
      | patch([0 0 1 1], [0 0.075 0.075 0], [230/255 0/255 0/255])
      | patch([0 0 1 1], [0.025 0.05 0.05 0.025], [150/255 0/255 0/255])
      | patch([0 0 1 1], [0 0.025 0.025 0], [0/255 0/255 0/255])
      | 
      | disp('dT');
  Out : Outport
  wires:
  IC/1 -> Switch1/1
  Max/1 -> Saturation/3(max)
  Min/1 -> Saturation/2(min)
  Data Type Conversion/1 -> Switch1/2
  Rst/1 -> Data Type Conversion/1
  Unit Delay/1 -> Switch1/3
  Product/1 -> Sum/2
  In/1 -> Product/1
  motohawk_delta_time/1 -> Product/2
  Switch1/1 -> Out/1, Sum/1
  Sum/1 -> Saturation/1(in)
  Saturation/1(out) -> Unit Delay/1

== system motohawk_engine_lib/O2A/Equivalence Ratio Perturbation/Hysteresis ==
  note: Hi & !Lo => Hi
      | Lo & !Hi => Lo
      | Otherwise, Hold
  Hi : Inport
  Lo : Inport  Port=2
  Combinatorial  Logic : CombinatorialLogic  TruthTable=[0 0;0 1;1 1;0 0]
  Demux : Demux  Outputs=2
  Mux : Mux  Inputs=2
  Switch1 : Switch  Threshold=0.5  SaturateOnIntegerOverflow=on  InputSameDT=on
  Unit Delay : UnitDelay  Orientation=left  SampleTime=-1
  "Out (Lo=0, Hi=1)" : Outport
  wires:
  Lo/1 -> Mux/2
  Hi/1 -> Mux/1
  Switch1/1 -> "Out (Lo=0, Hi=1)"/1, Unit Delay/1
  Unit Delay/1 -> Switch1/3
  Demux/2 -> Switch1/2
  Demux/1 -> Switch1/1
  Combinatorial  Logic/1 -> Demux/1
  Mux/1 -> Combinatorial  Logic/1

== system motohawk_engine_lib/Speed Density - MAP Referenced - Adaptive/Adapt Volumetric Efficiency/Adapt VolEff Map ==
  error : Inport
  Enable : EnablePort
  motohawk_adapt_table : MotoHawk_lib/Lookup Tables/motohawk_adapt_table  nam='VolEff'  typ=double  mode=Adapt between points
  wires:
  error/1 -> motohawk_adapt_table/1

== system motohawk_engine_lib/Speed Density - MAP Referenced - Adaptive/Adapt Volumetric Efficiency/Safe Divide ==
  X : Inport
  Inport : Inport  Port=2
  Constant : Constant  Value=0
  Relational Operator : RelationalOperator  Operator=~=  ZeroCross=off  InputSameDT=on
  Subsystem : Subsystem
  " " : Outport  InitialOutput=0
  wires:
  Constant/1 -> Relational Operator/1
  Relational Operator/1 -> Subsystem/Enable
  Subsystem/1(Out1) -> " "/1
  ? -> Relational Operator/2, Subsystem/2(In2)
  X/1 -> Subsystem/1(In1)

== system motohawk_engine_lib/Linear Sensor Characterization w Adapt/ADAPT SCALING/ADAPT HI/Store Current Position ==
  IN_FILT : Inport
  Enable : EnablePort
  Data Type Conversion2 : DataTypeConversion  OutDataTypeMode=uint16  SaturateOnIntegerOverflow=on  RndMeth=Zero
  motohawk_data_write : MotoHawk_lib/Data Storage Blocks/motohawk_data_write  source=Lookup By Name  structure=Scalar  operation=Write entire data structure at once  sz_vec=-1  sz_row=3  sz_col=2  typ=uint16  nam=[prefix 'Raw_Adpt_Hi']  checkNull=off  write_read_only=off  struct_inst_name='Struct1'
  wires:
  IN_FILT/1 -> Data Type Conversion2/1
  Data Type Conversion2/1 -> motohawk_data_write/1

== system motohawk_engine_lib/Linear Sensor Characterization w Adapt/ADAPT SCALING/ADAPT LO/Store Current Position ==
  IN_FILT : Inport
  Enable : EnablePort
  Data Type Conversion2 : DataTypeConversion  OutDataTypeMode=uint16  SaturateOnIntegerOverflow=on  RndMeth=Zero
  motohawk_data_write : MotoHawk_lib/Data Storage Blocks/motohawk_data_write  source=Lookup By Name  structure=Scalar  operation=Write entire data structure at once  sz_vec=-1  sz_row=3  sz_col=2  typ=uint16  nam=[prefix 'Raw_Adpt_Low']  checkNull=off  write_read_only=off  struct_inst_name='Struct1'
  wires:
  Data Type Conversion2/1 -> motohawk_data_write/1
  IN_FILT/1 -> Data Type Conversion2/1

== system motohawk_engine_lib/Model Fuel Puddle Mass/Enabled Tau-X Algorithm/Tau-X Fuel Model/[1/ (1 - X)] [Fdes - Mpud / T] ==
  Fdes [g/s] : Inport
  X [frac] : Inport  Port=2
  Tau [1/s] : Inport  Port=3
  Mpud [g] : Inport  Port=4
  Constant : Constant
  Product : Product  Inputs=*/  SaturateOnIntegerOverflow=on  InputSameDT=on
  Product1 : Product  Inputs=**  SaturateOnIntegerOverflow=on  InputSameDT=on
  Product2 : Product  Inputs=*/  SaturateOnIntegerOverflow=on  InputSameDT=on
  Sum : Sum  Inputs=|+-  SaturateOnIntegerOverflow=on  InputSameDT=on
  Sum1 : Sum  Inputs=|+-  SaturateOnIntegerOverflow=on  InputSameDT=on
  Finj [g/s] : Outport
  X_Mult : Outport  Port=2
  Tau_Ofst : Outport  Port=3
  wires:
  Constant/1 -> Product/1, Sum/1
  X [frac]/1 -> Sum/2
  Sum/1 -> Product/2
  Mpud [g]/1 -> Product2/1
  Tau [1/s]/1 -> Product2/2
  Fdes [g/s]/1 -> Sum1/1
  Product2/1 -> Tau_Ofst/1, Sum1/2
  Sum1/1 -> Product1/1  "Fdes - Mpud / T"
  Product/1 -> X_Mult/1, Product1/2  "1 / (1 - X)"
  Product1/1 -> Finj [g/s]/1

== system motohawk_engine_lib/Model Fuel Puddle Mass/Enabled Tau-X Algorithm/Tau-X Fuel Model/motohawk_TitleBlock ==

== system motohawk_engine_lib/Normalized Effective Combustion Chamber Temperature/Integrate an offset to ECT  Reset offset when engine is stopped./Integrator/Saturation ==
  note: Output 'In' when between Min and Max,
      | and saturate against limits otherwise.
  in : Inport
  min : Inport  Port=2
  max : Inport  Port=3
  MinMax : MinMax  Function=max  Inputs=2  ZeroCross=off  SaturateOnIntegerOverflow=on  InputSameDT=on
  MinMax1 : MinMax  Inputs=2  ZeroCross=off  SaturateOnIntegerOverflow=on  InputSameDT=on
  out : Outport
  wires:
  MinMax1/1 -> out/1
  max/1 -> MinMax1/2
  min/1 -> MinMax/2
  in/1 -> MinMax/1
  MinMax/1 -> MinMax1/1

== system motohawk_engine_lib/Speed Density - MAP Referenced - Adaptive/Adapt Volumetric Efficiency/Safe Divide/Subsystem ==
  In1 : Inport
  In2 : Inport  Port=2
  Enable : EnablePort
  Product1 : Product  Inputs=*/  SaturateOnIntegerOverflow=on  InputSameDT=on
  Out1 : Outport  InitialOutput=0
  wires:
  In2/1 -> Product1/2
  Product1/1 -> Out1/1
  In1/1 -> Product1/1

== stateflow chart Idle Governor/Idle State Determination/Idle State Machine ==
  state OffIdle
    /en: IdleState = 3;
  state Flaring
    /en: IdleState = 1;
  state OnIdle
    /en: IdleState = 2;
  (default) -> Flaring
  Flaring -> OffIdle [order 1] : [ThrPosHigh || !IdleEnable]
  OffIdle -> OnIdle : [RPMLow && ThrPosLow && IdleEnable]
  Flaring -> OnIdle [order 2] : [RPMFalling && ThrPosLow]
  OnIdle -> OffIdle : [ThrPosHigh || !IdleEnable]
  data: IdleEnable input boolean; RPMFalling input boolean; RPMLow input boolean; ThrPosLow input boolean; ThrPosHigh input boolean; IdleState output uint8
